simulink model "Part1_2"  (R2017a)
settings: Solver=VariableStepAuto  StartTime=0.0  StopTime=10  RelTol=1e-3
libraries: dsparch4 x2, commchan3 x1
settings Model: Creator=mhuynh7  LastModifiedBy=mhuynh7

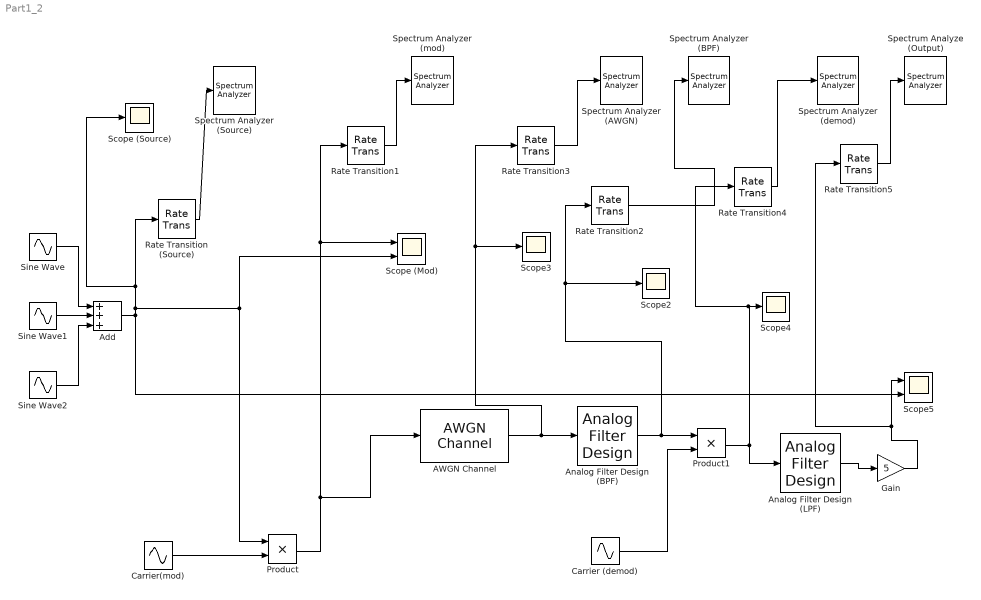
== system Part1_2 ==
  AWGN Channel : commchan3/AWGN Channel  InputProcessing=Columns as channels (frame based)  seed=randseed  noiseMode=Variance from mask  EbNodB=10  EsNodB=10  SNRdB=10  bitsPerSym=1  Ps=1  Tsym=1  variance=0.01
  Add : Sum  Inputs=+++
  Analog Filter Design (BPF) : dsparch4/Analog Filter Design  method=Butterworth  filttype=Bandpass  N=8  Wlo=14300*2*pi  Whi=15800*2*pi  Rp=2  Rs=40
  Analog Filter Design (LPF) : dsparch4/Analog Filter Design  method=Butterworth  filttype=Lowpass  N=8  Wlo=800*2*pi  Whi=80  Rp=2  Rs=40
  Carrier (demod) : Sin  Frequency=30000*pi  Phase=pi/2  SampleTime=0
  Carrier(mod) : Sin  Frequency=30000*pi  Phase=pi/2  SampleTime=0
  Gain : Gain  Gain=5
  Product : Product
  Product1 : Product
  Rate Transition (Source) : RateTransition  OutPortSampleTime=1/50000
  Rate Transition{1..5} (5 alike) : RateTransition  OutPortSampleTime=1/50000
  Scope (Mod) : Scope  NumInputPorts=2
  Scope (Source) : Scope
  Scope2 : Scope
  Scope3 : Scope
  Scope4 : Scope
  Scope5 : Scope  NumInputPorts=2
  Sine Wave : Sin  Frequency=1000*pi  SampleTime=0
  Sine Wave1 : Sin  Amplitude=3  Frequency=600*pi  SampleTime=0
  Sine Wave2 : Sin  Amplitude=1.5  Frequency=1200*pi  SampleTime=0
  Spectrum Analyze (Output) : SpectrumAnalyzer
  Spectrum Analyzer (AWGN) : SpectrumAnalyzer
  Spectrum Analyzer (BPF) : SpectrumAnalyzer
  Spectrum Analyzer (Source) : SpectrumAnalyzer
  Spectrum Analyzer (demod) : SpectrumAnalyzer
  Spectrum Analyzer (mod) : SpectrumAnalyzer
  wires:
  Sine Wave/1 -> Add/1
  Sine Wave1/1 -> Add/2
  Sine Wave2/1 -> Add/3
  Add/1 -> Scope (Mod)/2, Product/1, Rate Transition (Source)/1, Scope (Source)/1, Scope5/2
  Carrier(mod)/1 -> Product/2
  Rate Transition (Source)/1 -> Spectrum Analyzer (Source)/1
  Product/1 -> AWGN Channel/1, Rate Transition1/1, Scope (Mod)/1
  Rate Transition1/1 -> Spectrum Analyzer (mod)/1
  AWGN Channel/1 -> Scope3/1, Rate Transition3/1, Analog Filter Design (BPF)/1
  Analog Filter Design (BPF)/1 -> Rate Transition2/1, Scope2/1, Product1/1
  Carrier (demod)/1 -> Product1/2
  Product1/1 -> Analog Filter Design (LPF)/1, Rate Transition4/1, Scope4/1
  Analog Filter Design (LPF)/1 -> Gain/1
  Gain/1 -> Rate Transition5/1, Scope5/1
  Rate Transition5/1 -> Spectrum Analyze (Output)/1
  Rate Transition4/1 -> Spectrum Analyzer (demod)/1
  Rate Transition3/1 -> Spectrum Analyzer (AWGN)/1
  Rate Transition2/1 -> Spectrum Analyzer (BPF)/1
